simulink library "gim"  (Simulink 8.1)
settings: Solver=ode45  StartTime=0.0  StopTime=10.0  RelTol=1e-3
undefined symbols (not defined in the file or in its folder): FALSE, KIFO_ACCRelSpeedNoTargets_kph, KIFO_ACCXPositionNoTargets_m, KIFO_LongAccelNoTargets_mps2, KIFO_RelSpeedNoTargets_kph, KIFO_TargetIdNoTargets_num, KIFO_XPositionNoTargets_m, KIFO_YPositionNoTargets_m, TRUE, ZERO_INT
libraries: hcu_lib x4
settings Model: Creator=xsellart  LastModifiedBy=AT015555

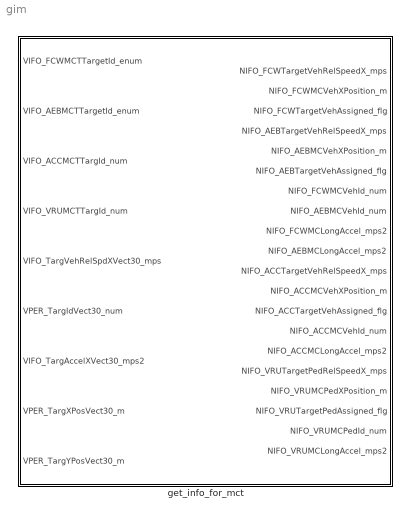
== system gim ==
  get_info_for_mct : Subsystem

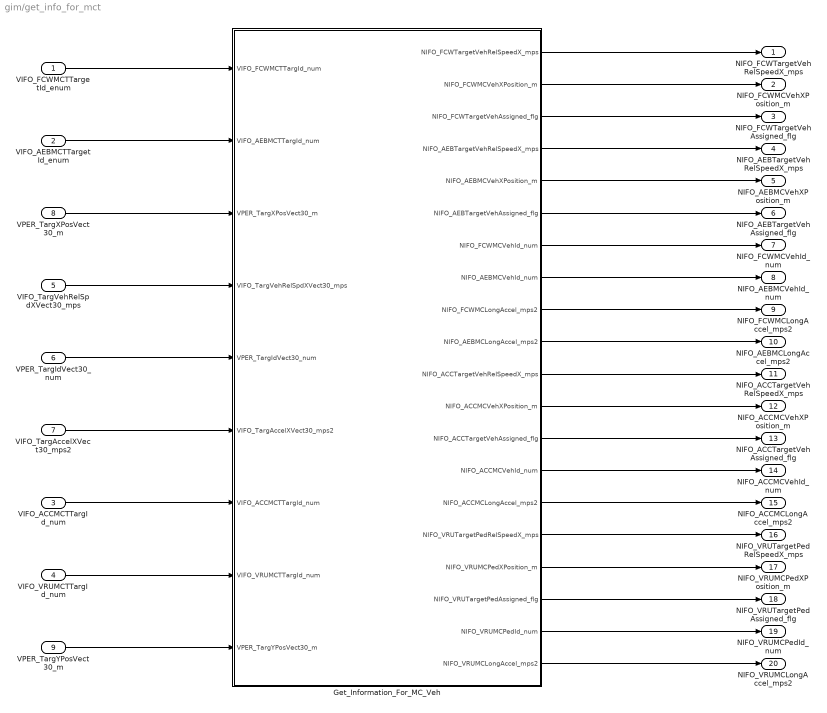
== system gim/get_info_for_mct ==
  VIFO_FCWMCTTargetId_enum : Inport
  VIFO_AEBMCTTargetId_enum : Inport  Port=2
  VIFO_ACCMCTTargId_num : Inport  Port=3
  VIFO_VRUMCTTargId_num : Inport  Port=4
  VIFO_TargVehRelSpdXVect30_mps : Inport  Port=5
  VPER_TargIdVect30_num : Inport  Port=6
  VIFO_TargAccelXVect30_mps2 : Inport  Port=7
  VPER_TargXPosVect30_m : Inport  Port=8
  VPER_TargYPosVect30_m : Inport  Port=9
  Get_Information_For_MC_Veh : Subsystem
  NIFO_FCWTargetVehRelSpeedX_mps : Outport
  NIFO_FCWMCVehXPosition_m : Outport  Port=2
  NIFO_FCWTargetVehAssigned_flg : Outport  Port=3
  NIFO_AEBTargetVehRelSpeedX_mps : Outport  Port=4
  NIFO_AEBMCVehXPosition_m : Outport  Port=5
  NIFO_AEBTargetVehAssigned_flg : Outport  Port=6
  NIFO_FCWMCVehId_num : Outport  Port=7
  NIFO_AEBMCVehId_num : Outport  Port=8
  NIFO_FCWMCLongAccel_mps2 : Outport  Port=9
  NIFO_AEBMCLongAccel_mps2 : Outport  Port=10
  NIFO_ACCTargetVehRelSpeedX_mps : Outport  Port=11
  NIFO_ACCMCVehXPosition_m : Outport  Port=12
  NIFO_ACCTargetVehAssigned_flg : Outport  Port=13
  NIFO_ACCMCVehId_num : Outport  Port=14
  NIFO_ACCMCLongAccel_mps2 : Outport  Port=15
  NIFO_VRUTargetPedRelSpeedX_mps : Outport  Port=16
  NIFO_VRUMCPedXPosition_m : Outport  Port=17
  NIFO_VRUTargetPedAssigned_flg : Outport  Port=18
  NIFO_VRUMCPedId_num : Outport  Port=19
  NIFO_VRUMCLongAccel_mps2 : Outport  Port=20
  wires:
  Get_Information_For_MC_Veh/20(NIFO_VRUMCLongAccel_mps2) -> NIFO_VRUMCLongAccel_mps2/1
  Get_Information_For_MC_Veh/19(NIFO_VRUMCPedId_num) -> NIFO_VRUMCPedId_num/1
  Get_Information_For_MC_Veh/18(NIFO_VRUTargetPedAssigned_flg) -> NIFO_VRUTargetPedAssigned_flg/1
  Get_Information_For_MC_Veh/17(NIFO_VRUMCPedXPosition_m) -> NIFO_VRUMCPedXPosition_m/1
  Get_Information_For_MC_Veh/16(NIFO_VRUTargetPedRelSpeedX_mps) -> NIFO_VRUTargetPedRelSpeedX_mps/1
  VIFO_VRUMCTTargId_num/1 -> Get_Information_For_MC_Veh/8(VIFO_VRUMCTTargId_num)
  Get_Information_For_MC_Veh/15(NIFO_ACCMCLongAccel_mps2) -> NIFO_ACCMCLongAccel_mps2/1
  Get_Information_For_MC_Veh/14(NIFO_ACCMCVehId_num) -> NIFO_ACCMCVehId_num/1
  Get_Information_For_MC_Veh/13(NIFO_ACCTargetVehAssigned_flg) -> NIFO_ACCTargetVehAssigned_flg/1
  Get_Information_For_MC_Veh/12(NIFO_ACCMCVehXPosition_m) -> NIFO_ACCMCVehXPosition_m/1
  Get_Information_For_MC_Veh/11(NIFO_ACCTargetVehRelSpeedX_mps) -> NIFO_ACCTargetVehRelSpeedX_mps/1
  VIFO_ACCMCTTargId_num/1 -> Get_Information_For_MC_Veh/7(VIFO_ACCMCTTargId_num)
  Get_Information_For_MC_Veh/10(NIFO_AEBMCLongAccel_mps2) -> NIFO_AEBMCLongAccel_mps2/1
  Get_Information_For_MC_Veh/9(NIFO_FCWMCLongAccel_mps2) -> NIFO_FCWMCLongAccel_mps2/1
  VIFO_TargAccelXVect30_mps2/1 -> Get_Information_For_MC_Veh/6(VIFO_TargAccelXVect30_mps2)
  VIFO_FCWMCTTargetId_enum/1 -> Get_Information_For_MC_Veh/1(VIFO_FCWMCTTargId_num)
  Get_Information_For_MC_Veh/8(NIFO_AEBMCVehId_num) -> NIFO_AEBMCVehId_num/1
  Get_Information_For_MC_Veh/7(NIFO_FCWMCVehId_num) -> NIFO_FCWMCVehId_num/1
  VPER_TargIdVect30_num/1 -> Get_Information_For_MC_Veh/5(VPER_TargIdVect30_num)
  VIFO_AEBMCTTargetId_enum/1 -> Get_Information_For_MC_Veh/2(VIFO_AEBMCTTargId_num)
  Get_Information_For_MC_Veh/6(NIFO_AEBTargetVehAssigned_flg) -> NIFO_AEBTargetVehAssigned_flg/1
  Get_Information_For_MC_Veh/5(NIFO_AEBMCVehXPosition_m) -> NIFO_AEBMCVehXPosition_m/1
  Get_Information_For_MC_Veh/4(NIFO_AEBTargetVehRelSpeedX_mps) -> NIFO_AEBTargetVehRelSpeedX_mps/1
  VIFO_TargVehRelSpdXVect30_mps/1 -> Get_Information_For_MC_Veh/4(VIFO_TargVehRelSpdXVect30_mps)
  VPER_TargXPosVect30_m/1 -> Get_Information_For_MC_Veh/3(VPER_TargXPosVect30_m)
  Get_Information_For_MC_Veh/3(NIFO_FCWTargetVehAssigned_flg) -> NIFO_FCWTargetVehAssigned_flg/1
  Get_Information_For_MC_Veh/2(NIFO_FCWMCVehXPosition_m) -> NIFO_FCWMCVehXPosition_m/1
  Get_Information_For_MC_Veh/1(NIFO_FCWTargetVehRelSpeedX_mps) -> NIFO_FCWTargetVehRelSpeedX_mps/1
  VPER_TargYPosVect30_m/1 -> Get_Information_For_MC_Veh/9(VPER_TargYPosVect30_m)

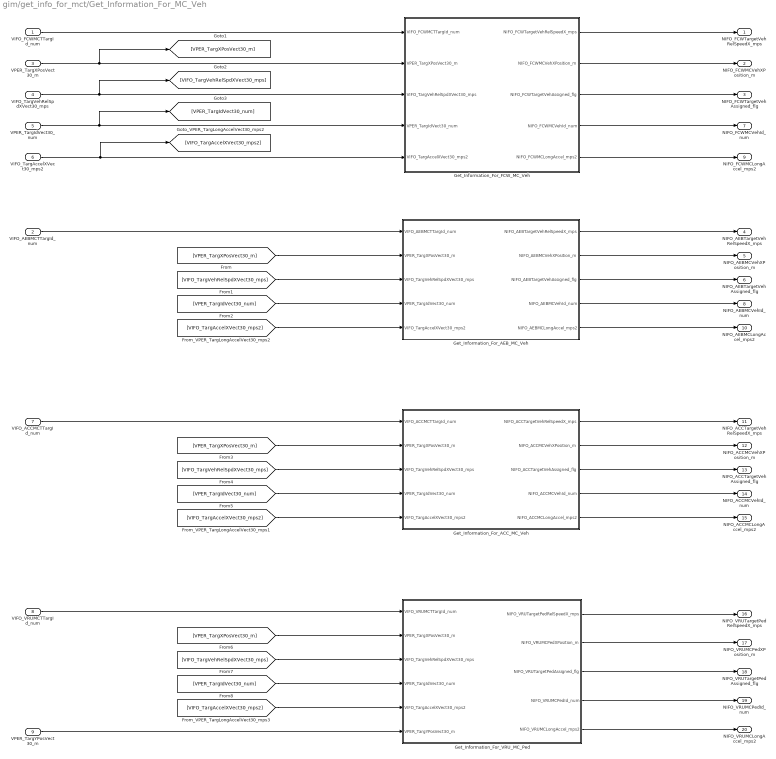
== system gim/get_info_for_mct/Get_Information_For_MC_Veh ==
  VIFO_FCWMCTTargId_num : Inport
  VIFO_AEBMCTTargId_num : Inport  Port=2
  VPER_TargXPosVect30_m : Inport  Port=3
  VIFO_TargVehRelSpdXVect30_mps : Inport  Port=4
  VPER_TargIdVect30_num : Inport  Port=5
  VIFO_TargAccelXVect30_mps2 : Inport  Port=6
  VIFO_ACCMCTTargId_num : Inport  Port=7
  VIFO_VRUMCTTargId_num : Inport  Port=8
  VPER_TargYPosVect30_m : Inport  Port=9
  Get_Information_For_ACC_MC_Veh : Subsystem
  Get_Information_For_AEB_MC_Veh : Subsystem
  Get_Information_For_FCW_MC_Veh : Subsystem
  Get_Information_For_VRU_MC_Ped : Subsystem
  NIFO_FCWTargetVehRelSpeedX_mps : Outport
  NIFO_FCWMCVehXPosition_m : Outport  Port=2
  NIFO_FCWTargetVehAssigned_flg : Outport  Port=3
  NIFO_AEBTargetVehRelSpeedX_mps : Outport  Port=4
  NIFO_AEBMCVehXPosition_m : Outport  Port=5
  NIFO_AEBTargetVehAssigned_flg : Outport  Port=6
  NIFO_FCWMCVehId_num : Outport  Port=7
  NIFO_AEBMCVehId_num : Outport  Port=8
  NIFO_FCWMCLongAccel_mps2 : Outport  Port=9
  NIFO_AEBMCLongAccel_mps2 : Outport  Port=10
  NIFO_ACCTargetVehRelSpeedX_mps : Outport  Port=11
  NIFO_ACCMCVehXPosition_m : Outport  Port=12
  NIFO_ACCTargetVehAssigned_flg : Outport  Port=13
  NIFO_ACCMCVehId_num : Outport  Port=14
  NIFO_ACCMCLongAccel_mps2 : Outport  Port=15
  NIFO_VRUTargetPedRelSpeedX_mps : Outport  Port=16
  NIFO_VRUMCPedXPosition_m : Outport  Port=17
  NIFO_VRUTargetPedAssigned_flg : Outport  Port=18
  NIFO_VRUMCPedId_num : Outport  Port=19
  NIFO_VRUMCLongAccel_mps2 : Outport  Port=20
  wires:
  Get_Information_For_VRU_MC_Ped/3(NIFO_VRUTargetPedAssigned_flg) -> NIFO_VRUTargetPedAssigned_flg/1
  Get_Information_For_VRU_MC_Ped/2(NIFO_VRUMCPedXPosition_m) -> NIFO_VRUMCPedXPosition_m/1
  Get_Information_For_VRU_MC_Ped/5(NIFO_VRUMCLongAccel_mps2) -> NIFO_VRUMCLongAccel_mps2/1
  Get_Information_For_VRU_MC_Ped/1(NIFO_VRUTargetPedRelSpeedX_mps) -> NIFO_VRUTargetPedRelSpeedX_mps/1
  [VIFO_TargAccelXVect30_mps2] -> Get_Information_For_VRU_MC_Ped/5(VIFO_TargAccelXVect30_mps2)
  [VPER_TargIdVect30_num] -> Get_Information_For_VRU_MC_Ped/4(VPER_TargIdVect30_num)
  [VIFO_TargVehRelSpdXVect30_mps] -> Get_Information_For_VRU_MC_Ped/3(VIFO_TargVehRelSpdXVect30_mps)
  [VPER_TargXPosVect30_m] -> Get_Information_For_VRU_MC_Ped/2(VPER_TargXPosVect30_m)
  VIFO_VRUMCTTargId_num/1 -> Get_Information_For_VRU_MC_Ped/1(VIFO_VRUMCTTargId_num)
  Get_Information_For_ACC_MC_Veh/5(NIFO_ACCMCLongAccel_mps2) -> NIFO_ACCMCLongAccel_mps2/1
  [VIFO_TargAccelXVect30_mps2] -> Get_Information_For_ACC_MC_Veh/5(VIFO_TargAccelXVect30_mps2)
  Get_Information_For_ACC_MC_Veh/4(NIFO_ACCMCVehId_num) -> NIFO_ACCMCVehId_num/1
  [VPER_TargIdVect30_num] -> Get_Information_For_ACC_MC_Veh/4(VPER_TargIdVect30_num)
  Get_Information_For_ACC_MC_Veh/3(NIFO_ACCTargetVehAssigned_flg) -> NIFO_ACCTargetVehAssigned_flg/1
  Get_Information_For_ACC_MC_Veh/2(NIFO_ACCMCVehXPosition_m) -> NIFO_ACCMCVehXPosition_m/1
  Get_Information_For_ACC_MC_Veh/1(NIFO_ACCTargetVehRelSpeedX_mps) -> NIFO_ACCTargetVehRelSpeedX_mps/1
  [VIFO_TargVehRelSpdXVect30_mps] -> Get_Information_For_ACC_MC_Veh/3(VIFO_TargVehRelSpdXVect30_mps)
  [VPER_TargXPosVect30_m] -> Get_Information_For_ACC_MC_Veh/2(VPER_TargXPosVect30_m)
  VIFO_ACCMCTTargId_num/1 -> Get_Information_For_ACC_MC_Veh/1(VIFO_ACCMCTTargId_num)
  Get_Information_For_AEB_MC_Veh/5(NIFO_AEBMCLongAccel_mps2) -> NIFO_AEBMCLongAccel_mps2/1
  [VIFO_TargAccelXVect30_mps2] -> Get_Information_For_AEB_MC_Veh/5(VIFO_TargAccelXVect30_mps2)
  Get_Information_For_FCW_MC_Veh/5(NIFO_FCWMCLongAccel_mps2) -> NIFO_FCWMCLongAccel_mps2/1
  VIFO_TargAccelXVect30_mps2/1 -> Get_Information_For_FCW_MC_Veh/5(VIFO_TargAccelXVect30_mps2), [VIFO_TargAccelXVect30_mps2]
  Get_Information_For_AEB_MC_Veh/4(NIFO_AEBMCVehId_num) -> NIFO_AEBMCVehId_num/1
  [VPER_TargIdVect30_num] -> Get_Information_For_AEB_MC_Veh/4(VPER_TargIdVect30_num)
  Get_Information_For_FCW_MC_Veh/4(NIFO_FCWMCVehId_num) -> NIFO_FCWMCVehId_num/1
  VPER_TargIdVect30_num/1 -> Get_Information_For_FCW_MC_Veh/4(VPER_TargIdVect30_num), [VPER_TargIdVect30_num]
  Get_Information_For_AEB_MC_Veh/3(NIFO_AEBTargetVehAssigned_flg) -> NIFO_AEBTargetVehAssigned_flg/1
  Get_Information_For_AEB_MC_Veh/2(NIFO_AEBMCVehXPosition_m) -> NIFO_AEBMCVehXPosition_m/1
  Get_Information_For_AEB_MC_Veh/1(NIFO_AEBTargetVehRelSpeedX_mps) -> NIFO_AEBTargetVehRelSpeedX_mps/1
  [VIFO_TargVehRelSpdXVect30_mps] -> Get_Information_For_AEB_MC_Veh/3(VIFO_TargVehRelSpdXVect30_mps)
  [VPER_TargXPosVect30_m] -> Get_Information_For_AEB_MC_Veh/2(VPER_TargXPosVect30_m)
  VIFO_AEBMCTTargId_num/1 -> Get_Information_For_AEB_MC_Veh/1(VIFO_AEBMCTTargId_num)
  Get_Information_For_FCW_MC_Veh/3(NIFO_FCWTargetVehAssigned_flg) -> NIFO_FCWTargetVehAssigned_flg/1
  Get_Information_For_FCW_MC_Veh/2(NIFO_FCWMCVehXPosition_m) -> NIFO_FCWMCVehXPosition_m/1
  Get_Information_For_FCW_MC_Veh/1(NIFO_FCWTargetVehRelSpeedX_mps) -> NIFO_FCWTargetVehRelSpeedX_mps/1
  VIFO_TargVehRelSpdXVect30_mps/1 -> Get_Information_For_FCW_MC_Veh/3(VIFO_TargVehRelSpdXVect30_mps), [VIFO_TargVehRelSpdXVect30_mps]
  VPER_TargXPosVect30_m/1 -> Get_Information_For_FCW_MC_Veh/2(VPER_TargXPosVect30_m), [VPER_TargXPosVect30_m]
  VIFO_FCWMCTTargId_num/1 -> Get_Information_For_FCW_MC_Veh/1(VIFO_FCWMCTTargId_num)
  Get_Information_For_VRU_MC_Ped/4(NIFO_VRUMCPedId_num) -> NIFO_VRUMCPedId_num/1
  VPER_TargYPosVect30_m/1 -> Get_Information_For_VRU_MC_Ped/6(VPER_TargYPosVect30_m)

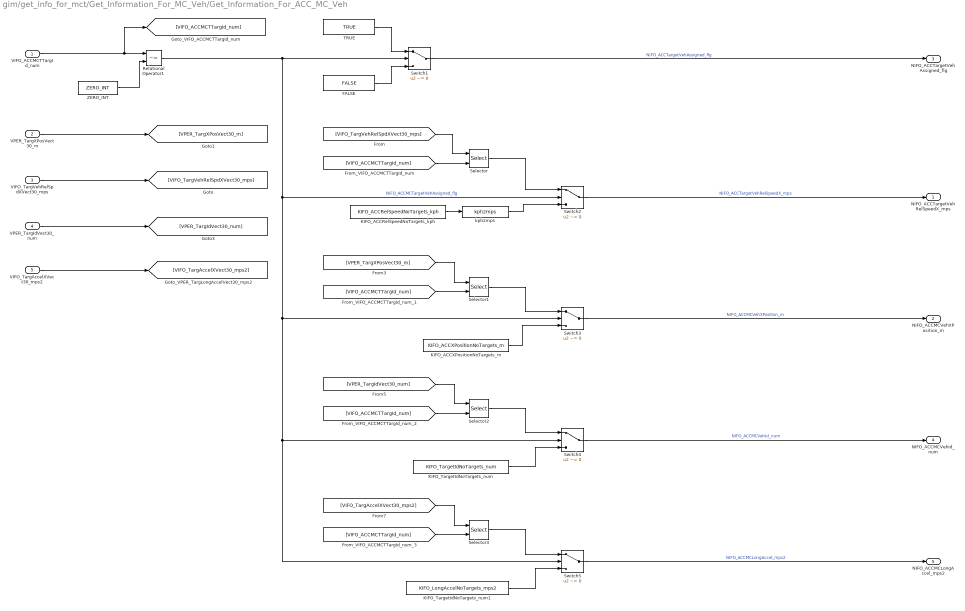
== system gim/get_info_for_mct/Get_Information_For_MC_Veh/Get_Information_For_ACC_MC_Veh ==
  VIFO_ACCMCTTargId_num : Inport
  VPER_TargXPosVect30_m : Inport  Port=2
  VIFO_TargVehRelSpdXVect30_mps : Inport  Port=3
  VPER_TargIdVect30_num : Inport  Port=4
  VIFO_TargAccelXVect30_mps2 : Inport  Port=5
  FALSE : Constant  Value=FALSE
  KIFO_ACCRelSpeedNoTargets_kph : Constant  Value=KIFO_ACCRelSpeedNoTargets_kph
  KIFO_ACCXPositionNoTargets_m : Constant  Value=KIFO_ACCXPositionNoTargets_m
  KIFO_TargetIdNoTargets_num : Constant  Value=KIFO_TargetIdNoTargets_num
  KIFO_TargetIdNoTargets_num1 : Constant  Value=KIFO_LongAccelNoTargets_mps2
  Relational Operator1 : RelationalOperator  Operator=~=  OutDataTypeStr=boolean
  Selector{,1..3} (4 alike) : Selector  InputPortWidth=30  IndexOptions=Index vector (port)  Indices=[1 3]  OutputSizes=1
  Switch{1..5} (5 alike) : Switch  Criteria=u2 ~= 0
  TRUE : Constant  Value=TRUE
  ZERO_INT : Constant  Value=ZERO_INT
  kph2mps : hcu_lib/kph2mps
  NIFO_ACCTargetVehRelSpeedX_mps : Outport
  NIFO_ACCMCVehXPosition_m : Outport  Port=2
  NIFO_ACCTargetVehAssigned_flg : Outport  Port=3
  NIFO_ACCMCVehId_num : Outport  Port=4
  NIFO_ACCMCLongAccel_mps2 : Outport  Port=5
  wires:
  Switch3/1 -> NIFO_ACCMCVehXPosition_m/1  "NIFO_ACCMCVehXPosition_m"
  Selector/1 -> Switch2/1
  [VPER_TargXPosVect30_m] -> Selector1/1
  [VIFO_TargVehRelSpdXVect30_mps] -> Selector/1
  FALSE/1 -> Switch1/3
  Switch1/1 -> NIFO_ACCTargetVehAssigned_flg/1  "NIFO_ACCTargetVehAssigned_flg"
  TRUE/1 -> Switch1/1
  ZERO_INT/1 -> Relational Operator1/2
  KIFO_ACCXPositionNoTargets_m/1 -> Switch3/3
  Selector1/1 -> Switch3/1
  VPER_TargXPosVect30_m/1 -> [VPER_TargXPosVect30_m]
  Switch2/1 -> NIFO_ACCTargetVehRelSpeedX_mps/1  "NIFO_ACCTargetVehRelSpeedX_mps"
  [VIFO_ACCMCTTargId_num] -> Selector1/2
  [VIFO_ACCMCTTargId_num] -> Selector/2
  VIFO_TargVehRelSpdXVect30_mps/1 -> [VIFO_TargVehRelSpdXVect30_mps]
  VIFO_ACCMCTTargId_num/1 -> [VIFO_ACCMCTTargId_num], Relational Operator1/1
  KIFO_ACCRelSpeedNoTargets_kph/1 -> kph2mps/1
  VPER_TargIdVect30_num/1 -> [VPER_TargIdVect30_num]
  Switch4/1 -> NIFO_ACCMCVehId_num/1  "NIFO_ACCMCVehId_num"
  [VPER_TargIdVect30_num] -> Selector2/1
  KIFO_TargetIdNoTargets_num/1 -> Switch4/3
  Selector2/1 -> Switch4/1
  [VIFO_ACCMCTTargId_num] -> Selector2/2
  kph2mps/1 -> Switch2/3
  VIFO_TargAccelXVect30_mps2/1 -> [VIFO_TargAccelXVect30_mps2]
  Switch5/1 -> NIFO_ACCMCLongAccel_mps2/1  "NIFO_ACCMCLongAccel_mps2"
  [VIFO_TargAccelXVect30_mps2] -> Selector3/1
  KIFO_TargetIdNoTargets_num1/1 -> Switch5/3
  Selector3/1 -> Switch5/1
  [VIFO_ACCMCTTargId_num] -> Selector3/2
  Relational Operator1/1 -> Switch5/2, Switch4/2, Switch3/2, Switch2/2, Switch1/2  "NIFO_ACCMCTargetVehAssigned_flg"

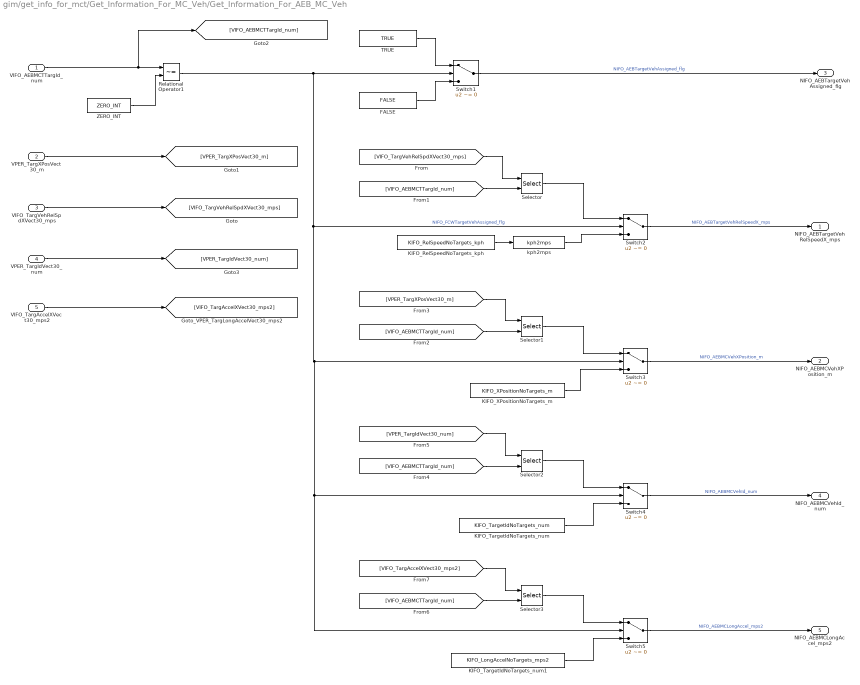
== system gim/get_info_for_mct/Get_Information_For_MC_Veh/Get_Information_For_AEB_MC_Veh ==
  VIFO_AEBMCTTargId_num : Inport
  VPER_TargXPosVect30_m : Inport  Port=2
  VIFO_TargVehRelSpdXVect30_mps : Inport  Port=3
  VPER_TargIdVect30_num : Inport  Port=4
  VIFO_TargAccelXVect30_mps2 : Inport  Port=5
  FALSE : Constant  Value=FALSE
  KIFO_RelSpeedNoTargets_kph : Constant  Value=KIFO_RelSpeedNoTargets_kph
  KIFO_TargetIdNoTargets_num : Constant  Value=KIFO_TargetIdNoTargets_num
  KIFO_TargetIdNoTargets_num1 : Constant  Value=KIFO_LongAccelNoTargets_mps2
  KIFO_XPositionNoTargets_m : Constant  Value=KIFO_XPositionNoTargets_m
  Relational Operator1 : RelationalOperator  Operator=~=  OutDataTypeStr=boolean
  Selector{,1..3} (4 alike) : Selector  InputPortWidth=30  IndexOptions=Index vector (port)  Indices=[1 3]  OutputSizes=1
  Switch{1..5} (5 alike) : Switch  Criteria=u2 ~= 0
  TRUE : Constant  Value=TRUE
  ZERO_INT : Constant  Value=ZERO_INT
  kph2mps : hcu_lib/kph2mps
  NIFO_AEBTargetVehRelSpeedX_mps : Outport
  NIFO_AEBMCVehXPosition_m : Outport  Port=2
  NIFO_AEBTargetVehAssigned_flg : Outport  Port=3
  NIFO_AEBMCVehId_num : Outport  Port=4
  NIFO_AEBMCLongAccel_mps2 : Outport  Port=5
  wires:
  Relational Operator1/1 -> Switch1/2, Switch2/2, Switch3/2, Switch4/2, Switch5/2  "NIFO_FCWTargetVehAssigned_flg"
  [VIFO_AEBMCTTargId_num] -> Selector3/2
  Selector3/1 -> Switch5/1
  KIFO_TargetIdNoTargets_num1/1 -> Switch5/3
  [VIFO_TargAccelXVect30_mps2] -> Selector3/1
  Switch5/1 -> NIFO_AEBMCLongAccel_mps2/1  "NIFO_AEBMCLongAccel_mps2"
  VIFO_TargAccelXVect30_mps2/1 -> [VIFO_TargAccelXVect30_mps2]
  kph2mps/1 -> Switch2/3
  [VIFO_AEBMCTTargId_num] -> Selector2/2
  Selector2/1 -> Switch4/1
  KIFO_TargetIdNoTargets_num/1 -> Switch4/3
  [VPER_TargIdVect30_num] -> Selector2/1
  Switch4/1 -> NIFO_AEBMCVehId_num/1  "NIFO_AEBMCVehId_num"
  VPER_TargIdVect30_num/1 -> [VPER_TargIdVect30_num]
  KIFO_RelSpeedNoTargets_kph/1 -> kph2mps/1
  VIFO_AEBMCTTargId_num/1 -> Relational Operator1/1, [VIFO_AEBMCTTargId_num]
  VIFO_TargVehRelSpdXVect30_mps/1 -> [VIFO_TargVehRelSpdXVect30_mps]
  [VIFO_AEBMCTTargId_num] -> Selector/2
  [VIFO_AEBMCTTargId_num] -> Selector1/2
  Switch2/1 -> NIFO_AEBTargetVehRelSpeedX_mps/1  "NIFO_AEBTargetVehRelSpeedX_mps"
  VPER_TargXPosVect30_m/1 -> [VPER_TargXPosVect30_m]
  Selector1/1 -> Switch3/1
  KIFO_XPositionNoTargets_m/1 -> Switch3/3
  ZERO_INT/1 -> Relational Operator1/2
  TRUE/1 -> Switch1/1
  Switch1/1 -> NIFO_AEBTargetVehAssigned_flg/1  "NIFO_AEBTargetVehAssigned_flg"
  FALSE/1 -> Switch1/3
  [VIFO_TargVehRelSpdXVect30_mps] -> Selector/1
  [VPER_TargXPosVect30_m] -> Selector1/1
  Selector/1 -> Switch2/1
  Switch3/1 -> NIFO_AEBMCVehXPosition_m/1  "NIFO_AEBMCVehXPosition_m"

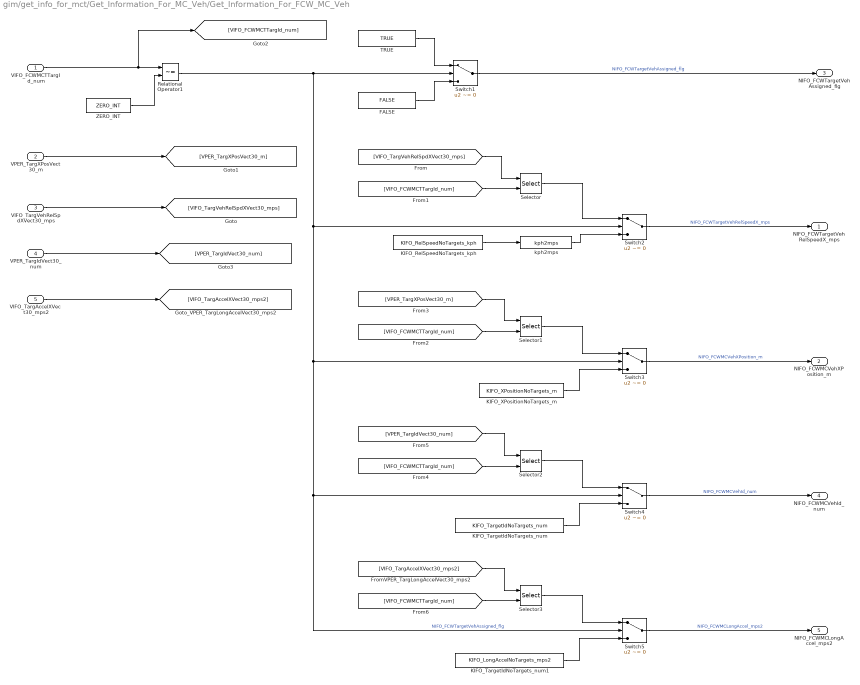
== system gim/get_info_for_mct/Get_Information_For_MC_Veh/Get_Information_For_FCW_MC_Veh ==
  VIFO_FCWMCTTargId_num : Inport
  VPER_TargXPosVect30_m : Inport  Port=2
  VIFO_TargVehRelSpdXVect30_mps : Inport  Port=3
  VPER_TargIdVect30_num : Inport  Port=4
  VIFO_TargAccelXVect30_mps2 : Inport  Port=5
  FALSE : Constant  Value=FALSE
  KIFO_RelSpeedNoTargets_kph : Constant  Value=KIFO_RelSpeedNoTargets_kph
  KIFO_TargetIdNoTargets_num : Constant  Value=KIFO_TargetIdNoTargets_num
  KIFO_TargetIdNoTargets_num1 : Constant  Value=KIFO_LongAccelNoTargets_mps2
  KIFO_XPositionNoTargets_m : Constant  Value=KIFO_XPositionNoTargets_m
  Relational Operator1 : RelationalOperator  Operator=~=  OutDataTypeStr=boolean
  Selector{,1..3} (4 alike) : Selector  InputPortWidth=30  IndexOptions=Index vector (port)  Indices=[1 3]  OutputSizes=1
  Switch{1..5} (5 alike) : Switch  Criteria=u2 ~= 0
  TRUE : Constant  Value=TRUE
  ZERO_INT : Constant  Value=ZERO_INT
  kph2mps : hcu_lib/kph2mps
  NIFO_FCWTargetVehRelSpeedX_mps : Outport
  NIFO_FCWMCVehXPosition_m : Outport  Port=2
  NIFO_FCWTargetVehAssigned_flg : Outport  Port=3
  NIFO_FCWMCVehId_num : Outport  Port=4
  NIFO_FCWMCLongAccel_mps2 : Outport  Port=5
  wires:
  Switch5/1 -> NIFO_FCWMCLongAccel_mps2/1  "NIFO_FCWMCLongAccel_mps2"
  [VIFO_TargAccelXVect30_mps2] -> Selector3/1
  KIFO_TargetIdNoTargets_num1/1 -> Switch5/3
  Selector3/1 -> Switch5/1
  [VIFO_FCWMCTTargId_num] -> Selector3/2
  Relational Operator1/1 -> Switch3/2, Switch4/2, Switch5/2, Switch2/2, Switch1/2  "NIFO_FCWTargetVehAssigned_flg"
  VIFO_TargAccelXVect30_mps2/1 -> [VIFO_TargAccelXVect30_mps2]
  kph2mps/1 -> Switch2/3
  Switch4/1 -> NIFO_FCWMCVehId_num/1  "NIFO_FCWMCVehId_num"
  [VPER_TargIdVect30_num] -> Selector2/1
  KIFO_TargetIdNoTargets_num/1 -> Switch4/3
  Selector2/1 -> Switch4/1
  [VIFO_FCWMCTTargId_num] -> Selector2/2
  VPER_TargIdVect30_num/1 -> [VPER_TargIdVect30_num]
  Switch3/1 -> NIFO_FCWMCVehXPosition_m/1  "NIFO_FCWMCVehXPosition_m"
  Selector/1 -> Switch2/1
  [VPER_TargXPosVect30_m] -> Selector1/1
  [VIFO_TargVehRelSpdXVect30_mps] -> Selector/1
  FALSE/1 -> Switch1/3
  Switch1/1 -> NIFO_FCWTargetVehAssigned_flg/1  "NIFO_FCWTargetVehAssigned_flg"
  TRUE/1 -> Switch1/1
  ZERO_INT/1 -> Relational Operator1/2
  KIFO_XPositionNoTargets_m/1 -> Switch3/3
  Selector1/1 -> Switch3/1
  VPER_TargXPosVect30_m/1 -> [VPER_TargXPosVect30_m]
  Switch2/1 -> NIFO_FCWTargetVehRelSpeedX_mps/1  "NIFO_FCWTargetVehRelSpeedX_mps"
  [VIFO_FCWMCTTargId_num] -> Selector1/2
  [VIFO_FCWMCTTargId_num] -> Selector/2
  VIFO_TargVehRelSpdXVect30_mps/1 -> [VIFO_TargVehRelSpdXVect30_mps]
  VIFO_FCWMCTTargId_num/1 -> [VIFO_FCWMCTTargId_num], Relational Operator1/1
  KIFO_RelSpeedNoTargets_kph/1 -> kph2mps/1

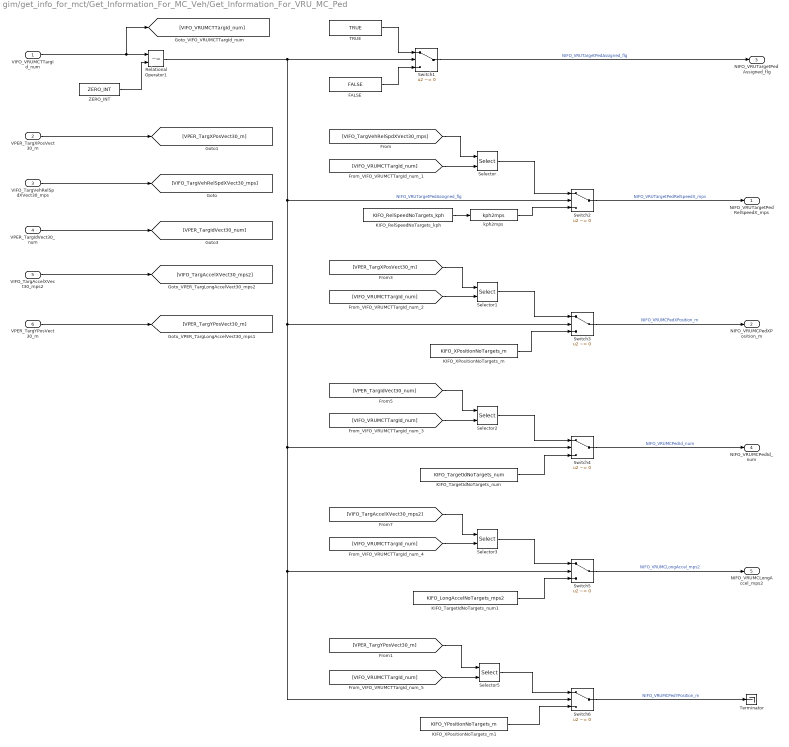
== system gim/get_info_for_mct/Get_Information_For_MC_Veh/Get_Information_For_VRU_MC_Ped ==
  VIFO_VRUMCTTargId_num : Inport
  VPER_TargXPosVect30_m : Inport  Port=2
  VIFO_TargVehRelSpdXVect30_mps : Inport  Port=3
  VPER_TargIdVect30_num : Inport  Port=4
  VIFO_TargAccelXVect30_mps2 : Inport  Port=5
  VPER_TargYPosVect30_m : Inport  Port=6
  FALSE : Constant  Value=FALSE
  KIFO_RelSpeedNoTargets_kph : Constant  Value=KIFO_RelSpeedNoTargets_kph
  KIFO_TargetIdNoTargets_num : Constant  Value=KIFO_TargetIdNoTargets_num
  KIFO_TargetIdNoTargets_num1 : Constant  Value=KIFO_LongAccelNoTargets_mps2
  KIFO_XPositionNoTargets_m : Constant  Value=KIFO_XPositionNoTargets_m
  KIFO_XPositionNoTargets_m1 : Constant  Value=KIFO_YPositionNoTargets_m
  Relational Operator1 : RelationalOperator  Operator=~=  OutDataTypeStr=boolean
  Selector{,1..3,5} (5 alike) : Selector  InputPortWidth=30  IndexOptions=Index vector (port)  Indices=[1 3]  OutputSizes=1
  Switch{1..6} (6 alike) : Switch  Criteria=u2 ~= 0
  TRUE : Constant  Value=TRUE
  Terminator : Terminator
  ZERO_INT : Constant  Value=ZERO_INT
  kph2mps : hcu_lib/kph2mps
  NIFO_VRUTargetPedRelSpeedX_mps : Outport
  NIFO_VRUMCPedXPosition_m : Outport  Port=2
  NIFO_VRUTargetPedAssigned_flg : Outport  Port=3
  NIFO_VRUMCPedId_num : Outport  Port=4
  NIFO_VRUMCLongAccel_mps2 : Outport  Port=5
  wires:
  Switch3/1 -> NIFO_VRUMCPedXPosition_m/1  "NIFO_VRUMCPedXPosition_m"
  Selector/1 -> Switch2/1
  [VPER_TargXPosVect30_m] -> Selector1/1
  [VIFO_TargVehRelSpdXVect30_mps] -> Selector/1
  FALSE/1 -> Switch1/3
  Switch1/1 -> NIFO_VRUTargetPedAssigned_flg/1  "NIFO_VRUTargetPedAssigned_flg"
  TRUE/1 -> Switch1/1
  ZERO_INT/1 -> Relational Operator1/2
  KIFO_XPositionNoTargets_m/1 -> Switch3/3
  Selector1/1 -> Switch3/1
  VPER_TargXPosVect30_m/1 -> [VPER_TargXPosVect30_m]
  Switch2/1 -> NIFO_VRUTargetPedRelSpeedX_mps/1  "NIFO_VRUTargetPedRelSpeedX_mps"
  [VIFO_VRUMCTTargId_num] -> Selector1/2
  [VIFO_VRUMCTTargId_num] -> Selector/2
  VIFO_TargVehRelSpdXVect30_mps/1 -> [VIFO_TargVehRelSpdXVect30_mps]
  VIFO_VRUMCTTargId_num/1 -> [VIFO_VRUMCTTargId_num], Relational Operator1/1
  KIFO_RelSpeedNoTargets_kph/1 -> kph2mps/1
  VPER_TargIdVect30_num/1 -> [VPER_TargIdVect30_num]
  Switch4/1 -> NIFO_VRUMCPedId_num/1  "NIFO_VRUMCPedId_num"
  [VPER_TargIdVect30_num] -> Selector2/1
  KIFO_TargetIdNoTargets_num/1 -> Switch4/3
  Selector2/1 -> Switch4/1
  [VIFO_VRUMCTTargId_num] -> Selector2/2
  kph2mps/1 -> Switch2/3
  VIFO_TargAccelXVect30_mps2/1 -> [VIFO_TargAccelXVect30_mps2]
  Switch5/1 -> NIFO_VRUMCLongAccel_mps2/1  "NIFO_VRUMCLongAccel_mps2"
  [VIFO_TargAccelXVect30_mps2] -> Selector3/1
  KIFO_TargetIdNoTargets_num1/1 -> Switch5/3
  Selector3/1 -> Switch5/1
  [VIFO_VRUMCTTargId_num] -> Selector3/2
  Relational Operator1/1 -> Switch6/2, Switch5/2, Switch4/2, Switch3/2, Switch2/2, Switch1/2  "NIFO_VRUTargetPedAssigned_flg"
  VPER_TargYPosVect30_m/1 -> [VPER_TargYPosVect30_m]
  [VPER_TargYPosVect30_m] -> Selector5/1
  [VIFO_VRUMCTTargId_num] -> Selector5/2
  Selector5/1 -> Switch6/1
  KIFO_XPositionNoTargets_m1/1 -> Switch6/3
  Switch6/1 -> Terminator/1  "NIFO_VRUMCPedYPosition_m"
